simulink model "MPC_Controller"  (R2023b)
settings: Solver=VariableStepAuto  StartTime=0.0  StopTime=20  RelTol=1e-3
settings Model: Creator=patel  LastModifiedBy=patel

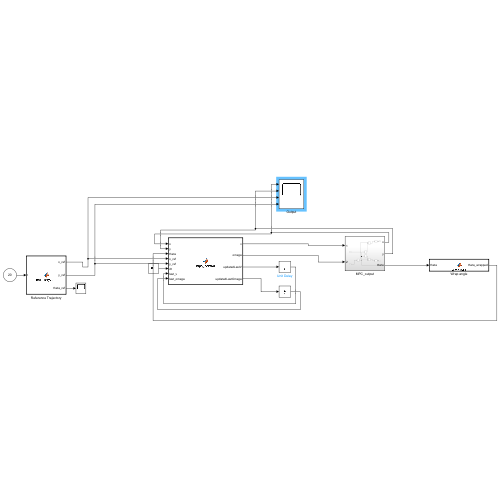
[thumbnail: Simulink's stored preview of the top-level diagram]
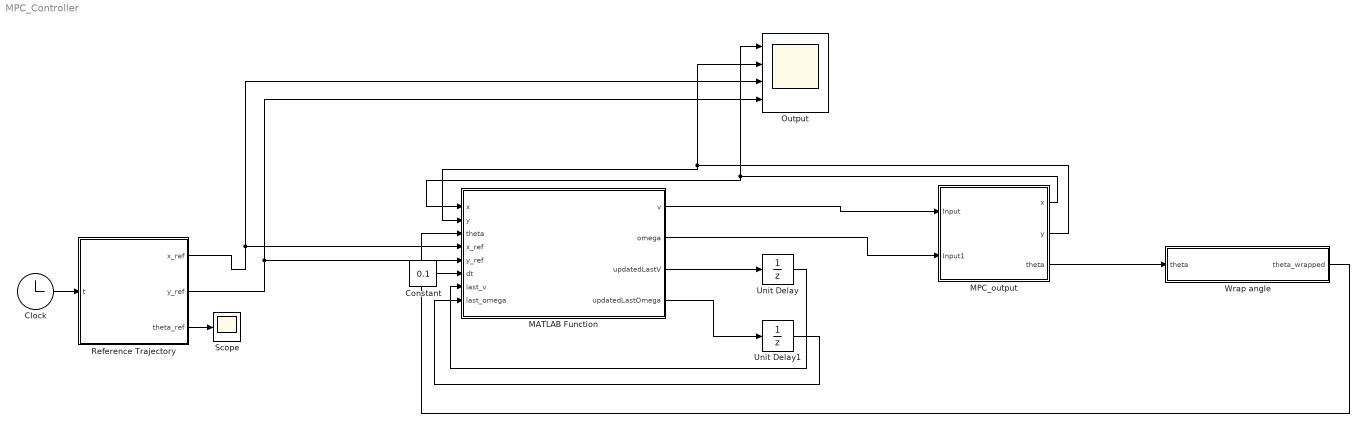
== system MPC_Controller ==
  Clock : Clock
      settings: Decimation=20
  Constant : Constant  Value=0.1
  MATLAB Function : MATLAB Function  TreatAsAtomicUnit=on
  MPC_output : Subsystem
  Output : Scope  NumInputPorts=4
  Reference Trajectory : MATLAB Function  TreatAsAtomicUnit=on
  Scope : Scope
  Unit Delay : UnitDelay  SampleTime=-1  HasFrameUpgradeWarning=on
  Unit Delay1 : UnitDelay  SampleTime=-1  HasFrameUpgradeWarning=on
  Wrap angle : MATLAB Function  TreatAsAtomicUnit=on
  wires:
  MPC_output/2(y) -> MATLAB Function/2(y), Output/2
  Clock/1 -> Reference Trajectory/1(t)
  MATLAB Function/1(v) -> MPC_output/1(Input)
  Constant/1 -> MATLAB Function/6(dt)
  MATLAB Function/2(omega) -> MPC_output/2(Input1)
  Reference Trajectory/3(theta_ref) -> Scope/1
  Reference Trajectory/1(x_ref) -> MATLAB Function/4(x_ref), Output/3
  Wrap angle/1(theta_wrapped) -> MATLAB Function/3(theta)
  MATLAB Function/3(updatedLastV) -> Unit Delay/1
  Reference Trajectory/2(y_ref) -> MATLAB Function/5(y_ref), Output/4
  MPC_output/1(x) -> MATLAB Function/1(x), Output/1
  Unit Delay/1 -> MATLAB Function/7(last_v)
  MPC_output/3(theta) -> Wrap angle/1(theta)
  MATLAB Function/4(updatedLastOmega) -> Unit Delay1/1
  Unit Delay1/1 -> MATLAB Function/8(last_omega)

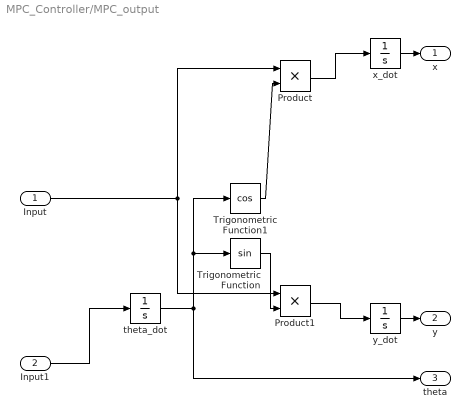
== system MPC_Controller/MPC_output ==
  Input : Inport
  Input1 : Inport  Port=2
  Product : Product
  Product1 : Product
  Trigonometric Function : Trigonometry
  Trigonometric Function1 : Trigonometry  Operator=cos
  theta_dot : Integrator
  x_dot : Integrator
  y_dot : Integrator
  x : Outport
  y : Outport  Port=2
  theta : Outport  Port=3
  wires:
  theta_dot/1 -> theta/1, Trigonometric Function1/1, Trigonometric Function/1
  Product/1 -> x_dot/1
  Input1/1 -> theta_dot/1
  Trigonometric Function1/1 -> Product/2
  Input/1 -> Product1/1, Product/1
  Trigonometric Function/1 -> Product1/2
  Product1/1 -> y_dot/1
  x_dot/1 -> x/1
  y_dot/1 -> y/1

== matlab function MPC_Controller/Reference Trajectory ==
  data: t input; x_ref output; y_ref output; theta_ref output
function [x_ref, y_ref, theta_ref] = trajectoryGen(t)
    radius = 5;
    omega_ref = 0.2;
    x_ref = radius * cos(omega_ref * t);
    y_ref = radius * sin(omega_ref * t);
    theta_ref = omega_ref * t + pi/2;
end

== matlab function MPC_Controller/Wrap angle ==
  data: theta input; theta_wrapped output
function theta_wrapped = wrapToPi(theta)
    theta_wrapped = mod(theta + pi, 2*pi) - pi;
end

== matlab function MPC_Controller/MATLAB Function ==
  data: x input; v output; y input; theta input; x_ref input; y_ref input; dt input; last_v input; omega output; updatedLastV output; last_omega input; updatedLastOmega output

function [v, omega, updatedLastV, updatedLastOmega] = mpc_control(x, y, theta, x_ref, y_ref, dt, last_v, last_omega)
%#codegen
robotState = [x; y; theta];
targetPoint = [x_ref; y_ref];
[v, omega, updatedLastV, updatedLastOmega] = MPCController(robotState, targetPoint, dt, last_v, last_omega);

function [best_v, best_omega, last_v, last_omega] = MPCController(robotState, targetPoint, dt, last_v, last_omega)
    % Unpack state
    x = robotState(1);
    y = robotState(2);
    theta = robotState(3);
    
    x_target = targetPoint(1);
    y_target = targetPoint(2);

    % MPC Parameters
    N = 10;  % Prediction horizon

    % Weights
    w_pos = 1.0;
    w_theta = 1.5;
    w_v = 0.1;
    w_omega = 0.2;

    % Control limits
    v_min = 0.2; v_max = 5.0;
    omega_min = -pi; omega_max = pi;

    % Discretized control space
    v_options = linspace(max(v_min, last_v - 0.5), min(v_max, last_v + 0.5), 5);
    omega_options = linspace(max(omega_min, last_omega - 0.5), min(omega_max, last_omega + 0.5), 7);

    % Initialize best control
    best_cost = inf;
    best_v = last_v;
    best_omega = last_omega;

    % Evaluate control sequences
    for vi = 1:length(v_options)
        for wi = 1:length(omega_options)
            v = v_options(vi);
            omega = omega_options(wi);

            pred_x = x;
            pred_y = y;
            pred_theta = theta;
            total_cost = 0;

            for i = 0:N-1
                % Predict next state
                pred_x = pred_x + v * cos(pred_theta) * dt;
                pred_y = pred_y + v * sin(pred_theta) * dt;
                pred_theta = pred_theta + omega * dt;

                % Compute errors
                pos_error = sqrt((x_target - pred_x)^2 + (y_target - pred_y)^2);
                desired_theta = atan2(y_target - pred_y, x_target - pred_x);
                theta_error = atan2(sin(desired_theta - pred_theta), cos(desired_theta - pred_theta));

                % Control smoothness
                v_change = abs(v - last_v);
                omega_change = abs(omega - last_omega);

                % Cost with discount
                step_cost = w_pos * pos_error + w_theta * abs(theta_error) + w_v * v_change + w_omega * omega_change;
                discount = 0.9 ^ i;
                total_cost = total_cost + discount * step_cost;
            end

            % Update best control
            if total_cost < best_cost
                best_cost = total_cost;
                best_v = v;
                best_omega = omega;
            end
        end
    end

    % Update memory for next step
    last_v = best_v;
    last_omega = best_omega;
end

end
